simulink model "mbed_disco_f407_counter_interrupt"  (R2015a)
settings: Solver=FixedStepDiscrete  SolverMode=SingleTasking  StartTime=0.0  StopTime=10.0  FixedStep=1  RelTol=1e-3
libraries: mbed_targets_stm_disco_f407 x2, simulink x1
settings Model: Creator=Stuv  LastModifiedBy=Stuv
settings OptimizationCC: OptimizeModelRefInitCode=on  LifeSpan=1
settings HardwareCC: ProdLargestAtomicInteger=Long  ProdLargestAtomicFloat=Double  ProdEndianess=LittleEndian  ProdHWDeviceType=ARM Compatible->ARM Cortex
settings RTWCC: SystemTargetFile=mbed.tlc  TemplateMakefile=mbed.tmf  Description=Mbed Target (Embedded Target)  TargetLang=C++
settings CodeAppCC: IgnoreCustomStorageClasses=off
settings STFCustomTargetCC: CombineOutputUpdateFcns=on  SupportContinuousTime=off  SupportVariableSizeSignals=off  SystemTargetFile=mbed.tlc
settings ERTTargetCC: SupportContinuousTime=off  SupportVariableSizeSignals=off  ERTCustomFileTemplate=mbed_file_process.tlc

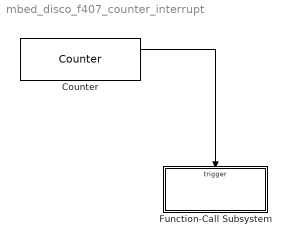
== system mbed_disco_f407_counter_interrupt ==
  Counter : mbed_targets_stm_disco_f407/Counter  TimerNumber=4  InputChannel=TI2 falling  TiPort=B  TiPin=7  TiPupd=PullUp  MaxCnt=6  Interrupt=interrupt + cnt output  RstEnable=off
  Function-Call Subsystem : Subsystem  TreatAsAtomicUnit=on
  wires:
  Counter/1 -> Function-Call Subsystem/Trigger

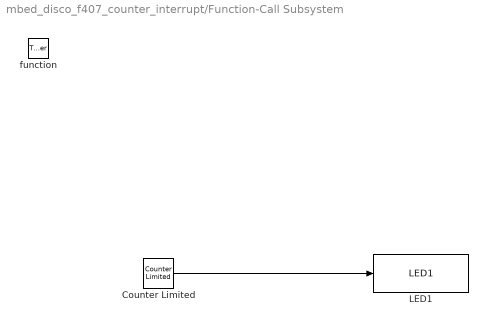
== system mbed_disco_f407_counter_interrupt/Function-Call Subsystem ==
  function : TriggerPort  TriggerType=function-call
  Counter Limited : simulink/Sources/Counter Limited  uplimit=1  tsamp=-1
  LED1 : mbed_targets_stm_disco_f407/LED1  Parameter1=0
  wires:
  Counter Limited/1 -> LED1/1
